simulink model "avarge"  (R2021a)
settings: Solver=FixedStepDiscrete  StartTime=0.0  StopTime=10.0  RelTol=1e-3  EnableMultiTasking=on
values from neighbouring files (symbols this model uses):
  num = 7    [avarge_var.m]
settings Model: Creator=Rana  LastModifiedBy=Rana
settings DataIOCC: ReturnWorkspaceOutputs=off
settings OptimizationCC: DefaultParameterBehavior=Inlined  InlineInvariantSignals=on  EnableMemcpy=off  LifeSpan=1  EfficientTunableParamExpr=on
settings DebuggingCC: UnderspecifiedInitializationDetection=Classic  MergeDetectMultiDrivingBlocksExec=none  SFMachineParentedDataDiag=warning  ArithmeticOperatorsInVariantConditions=warning
settings ModelReferenceCC: PropagateSignalLabelsOutOfModel=off
settings SFSimCC: MATLABDynamicMemAlloc=off  CustomCodeUndefinedFunction=UseInterfaceOnly
settings RTWCC: SystemTargetFile=ert.tlc  GenCodeOnly=on  TemplateMakefile=ert_default_tmf  GenerateReport=on  IncludeHyperlinkInReport=on  LaunchReport=on  GenerateTraceInfo=on  GenerateTraceReport=on  GenerateTraceReportSl=on  GenerateTraceReportSf=on  GenerateTraceReportEml=on
settings CodeAppCC: ForceParamTrailComments=on  IgnoreCustomStorageClasses=off  OperatorAnnotations=on  SimulinkDataObjDesc=on  SFDataObjDesc=on  MATLABFcnDesc=on  InsertBlockDesc=on  StateflowObjectComments=on  MATLABSourceComments=on
settings ERTTargetCC: MultiwordLength=2048  GenerateSampleERTMain=on  InlinedParameterPlacement=NonHierarchical  ERTCustomFileTemplate=example_file_process.tlc

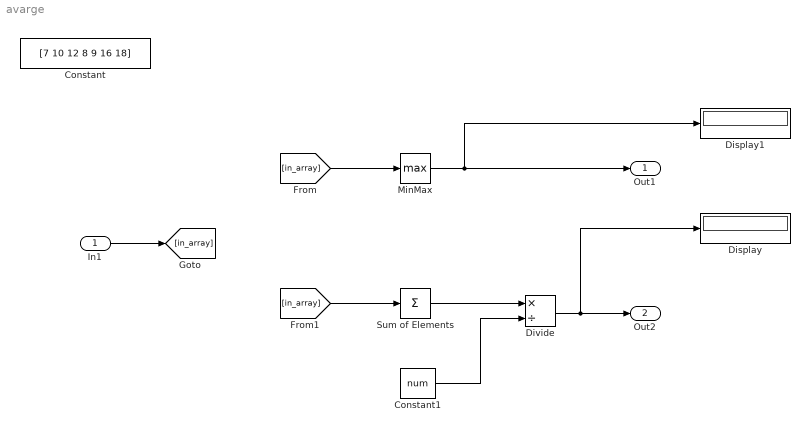
== system avarge ==
  In1 : Inport  PortDimensions=num
  Constant : Constant  Value=[7 10 12 8 9 16 18]
  Constant1 : Constant  Value=num
  Display : Display
  Display1 : Display
  Divide : Product  Inputs=*/
  MinMax : MinMax  Function=max
  Sum of Elements : Sum  Inputs=+
  Out1 : Outport  SignalName=max_min
  Out2 : Outport  Port=2  SignalName=avg
  wires:
  In1/1 -> [in_array]
  MinMax/1 -> Display1/1, Out1/1
  Sum of Elements/1 -> Divide/1
  Constant1/1 -> Divide/2
  Divide/1 -> Display/1, Out2/1
  [in_array] -> MinMax/1
  [in_array] -> Sum of Elements/1
